simulink model "PIPO"  (R2024a)
settings: Solver=VariableStepAuto  StartTime=0.0  StopTime=10.0  RelTol=1e-3
libraries: simulink_extras x14
settings Model: Creator=prath  LastModifiedBy=prath

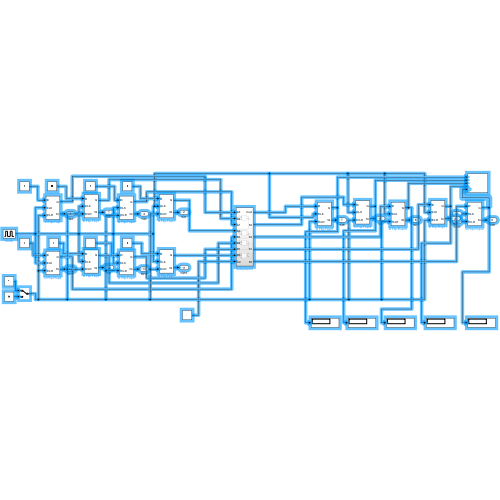
[thumbnail: Simulink's stored preview of the top-level diagram]
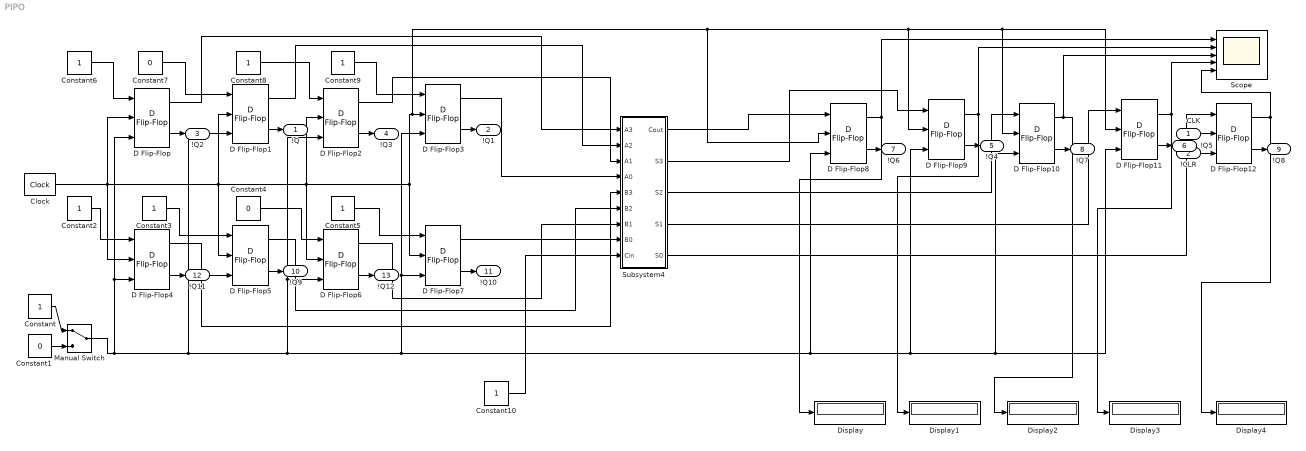
== system PIPO ==
  CLK : Inport
  !CLR : Inport  Port=2
  Clock : simulink_extras/Flip Flops/Clock  period=1
  Constant{,2..3,5..6,8..10} (8 alike) : Constant  OutDataTypeStr=boolean
  Constant1 : Constant  Value=0  OutDataTypeStr=boolean
  Constant4 : Constant  Value=0  OutDataTypeStr=boolean
  Constant7 : Constant  Value=0  OutDataTypeStr=boolean
  D Flip-Flop{,1..12} (13 alike) : simulink_extras/Flip Flops/D Flip-Flop
  Display{,1..4} (5 alike) : Display
  Manual Switch : ManualSwitch
  Scope : Scope  NumInputPorts=5
  Subsystem4 : Subsystem
  !Q : Outport
  !Q1 : Outport  Port=2
  !Q2 : Outport  Port=3
  !Q3 : Outport  Port=4
  !Q4 : Outport  Port=5
  !Q5 : Outport  Port=6
  !Q6 : Outport  Port=7
  !Q7 : Outport  Port=8
  !Q8 : Outport  Port=9
  !Q9 : Outport  Port=10
  !Q10 : Outport  Port=11
  !Q11 : Outport  Port=12
  !Q12 : Outport  Port=13
  wires:
  Subsystem4/5(S0) -> D Flip-Flop12/1
  D Flip-Flop/2 -> !Q2/1
  Constant/1 -> Manual Switch/1
  Constant7/1 -> D Flip-Flop1/1
  D Flip-Flop4/1 -> Subsystem4/5(B3)
  !CLR/1 -> D Flip-Flop12/3
  D Flip-Flop3/1 -> Subsystem4/4(A0)
  D Flip-Flop7/2 -> !Q10/1
  Constant8/1 -> D Flip-Flop2/1
  D Flip-Flop1/2 -> !Q/1
  D Flip-Flop/1 -> Subsystem4/1(A3)
  D Flip-Flop9/2 -> !Q4/1
  D Flip-Flop10/2 -> !Q7/1
  D Flip-Flop11/2 -> !Q5/1
  D Flip-Flop4/2 -> !Q11/1
  D Flip-Flop6/2 -> !Q12/1
  D Flip-Flop3/2 -> !Q1/1
  Constant5/1 -> D Flip-Flop7/1
  D Flip-Flop11/1 -> Scope/4, Display3/1
  Subsystem4/4(S1) -> D Flip-Flop11/1
  D Flip-Flop5/2 -> !Q9/1
  D Flip-Flop7/1 -> Subsystem4/8(B0)
  Subsystem4/1(Cout) -> D Flip-Flop8/1
  Constant9/1 -> D Flip-Flop3/1
  D Flip-Flop5/1 -> Subsystem4/6(B2)
  D Flip-Flop10/1 -> Scope/3, Display2/1
  Constant3/1 -> D Flip-Flop5/1
  D Flip-Flop1/1 -> Subsystem4/2(A2)
  CLK/1 -> D Flip-Flop12/2
  Constant4/1 -> D Flip-Flop6/1
  D Flip-Flop12/2 -> !Q8/1
  Subsystem4/3(S2) -> D Flip-Flop10/1
  D Flip-Flop8/1 -> Scope/1, Display/1
  D Flip-Flop8/2 -> !Q6/1
  Clock/1 -> D Flip-Flop4/2, D Flip-Flop/2, D Flip-Flop5/2, D Flip-Flop1/2, D Flip-Flop2/2, D Flip-Flop6/2, D Flip-Flop8/2, D Flip-Flop9/2, D Flip-Flop10/2, D Flip-Flop11/2, D Flip-Flop3/2, D Flip-Flop7/2
  Subsystem4/2(S3) -> D Flip-Flop9/1
  Constant2/1 -> D Flip-Flop4/1
  D Flip-Flop9/1 -> Scope/2, Display1/1
  Manual Switch/1 -> D Flip-Flop4/3, D Flip-Flop/3, D Flip-Flop5/3, D Flip-Flop1/3, D Flip-Flop2/3, D Flip-Flop6/3, D Flip-Flop8/3, D Flip-Flop9/3, D Flip-Flop10/3, D Flip-Flop11/3, D Flip-Flop7/3, D Flip-Flop3/3
  D Flip-Flop2/1 -> Subsystem4/3(A1)
  D Flip-Flop6/1 -> Subsystem4/7(B1)
  Constant6/1 -> D Flip-Flop/1
  Constant10/1 -> Subsystem4/9(Cin)
  Constant1/1 -> Manual Switch/2
  D Flip-Flop2/2 -> !Q3/1
  D Flip-Flop12/1 -> Scope/5, Display4/1

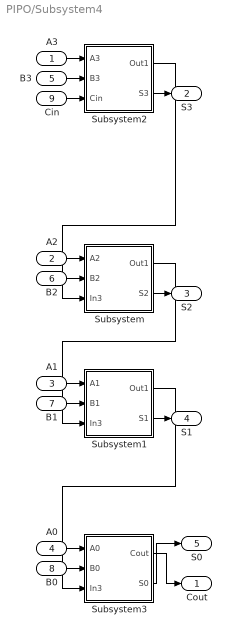
== system PIPO/Subsystem4 ==
  A3 : Inport
  A2 : Inport  Port=2
  A1 : Inport  Port=3
  A0 : Inport  Port=4
  B3 : Inport  Port=5
  B2 : Inport  Port=6
  B1 : Inport  Port=7
  B0 : Inport  Port=8
  Cin : Inport  Port=9
  Subsystem : Subsystem
  Subsystem1 : Subsystem
  Subsystem2 : Subsystem
  Subsystem3 : Subsystem
  Cout : Outport
  S3 : Outport  Port=2
  S2 : Outport  Port=3
  S1 : Outport  Port=4
  S0 : Outport  Port=5
  wires:
  Subsystem2/1(Out1) -> Subsystem/3(In3)
  Subsystem2/2(S3) -> S3/1
  B0/1 -> Subsystem3/2(B0)
  Subsystem1/1(Out1) -> Subsystem3/3(In3)
  Subsystem/1(Out1) -> Subsystem1/3(In3)
  Subsystem3/2(S0) -> S0/1
  A2/1 -> Subsystem/1(A2)
  Subsystem/2(S2) -> S2/1
  A0/1 -> Subsystem3/1(A0)
  B1/1 -> Subsystem1/2(B1)
  Subsystem3/1(Cout) -> Cout/1
  B2/1 -> Subsystem/2(B2)
  B3/1 -> Subsystem2/2(B3)
  Cin/1 -> Subsystem2/3(Cin)
  Subsystem1/2(S1) -> S1/1
  A3/1 -> Subsystem2/1(A3)
  A1/1 -> Subsystem1/1(A1)

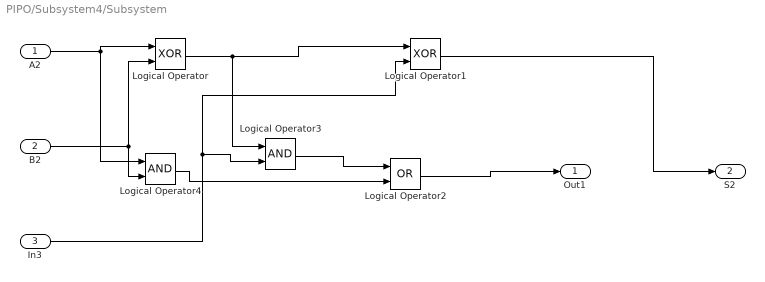
== system PIPO/Subsystem4/Subsystem ==
  A2 : Inport
  B2 : Inport  Port=2
  In3 : Inport  Port=3
  Logical Operator : Logic  Operator=XOR  AllPortsSameDT=off  OutDataTypeStr=boolean
  Logical Operator1 : Logic  Operator=XOR  AllPortsSameDT=off  OutDataTypeStr=boolean
  Logical Operator2 : Logic  Operator=OR  AllPortsSameDT=off  OutDataTypeStr=boolean
  Logical Operator3 : Logic  AllPortsSameDT=off  OutDataTypeStr=boolean
  Logical Operator4 : Logic  AllPortsSameDT=off  OutDataTypeStr=boolean
  Out1 : Outport
  S2 : Outport  Port=2
  wires:
  B2/1 -> Logical Operator/2, Logical Operator4/2
  Logical Operator/1 -> Logical Operator3/1, Logical Operator1/1
  In3/1 -> Logical Operator3/2, Logical Operator1/2
  Logical Operator3/1 -> Logical Operator2/1
  Logical Operator2/1 -> Out1/1
  A2/1 -> Logical Operator/1, Logical Operator4/1
  Logical Operator4/1 -> Logical Operator2/2
  Logical Operator1/1 -> S2/1

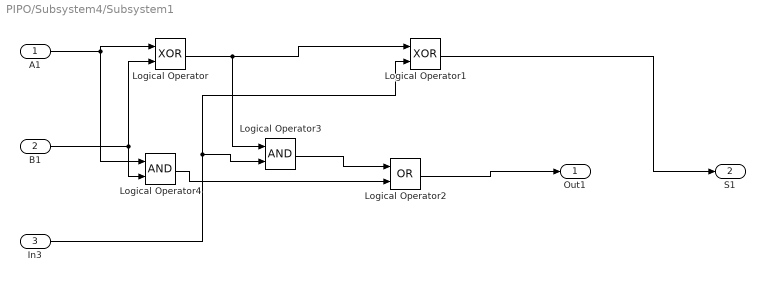
== system PIPO/Subsystem4/Subsystem1 ==
  A1 : Inport
  B1 : Inport  Port=2
  In3 : Inport  Port=3
  Logical Operator : Logic  Operator=XOR  AllPortsSameDT=off  OutDataTypeStr=boolean
  Logical Operator1 : Logic  Operator=XOR  AllPortsSameDT=off  OutDataTypeStr=boolean
  Logical Operator2 : Logic  Operator=OR  AllPortsSameDT=off  OutDataTypeStr=boolean
  Logical Operator3 : Logic  AllPortsSameDT=off  OutDataTypeStr=boolean
  Logical Operator4 : Logic  AllPortsSameDT=off  OutDataTypeStr=boolean
  Out1 : Outport
  S1 : Outport  Port=2
  wires:
  B1/1 -> Logical Operator/2, Logical Operator4/2
  Logical Operator/1 -> Logical Operator3/1, Logical Operator1/1
  In3/1 -> Logical Operator3/2, Logical Operator1/2
  Logical Operator3/1 -> Logical Operator2/1
  Logical Operator2/1 -> Out1/1
  A1/1 -> Logical Operator/1, Logical Operator4/1
  Logical Operator4/1 -> Logical Operator2/2
  Logical Operator1/1 -> S1/1

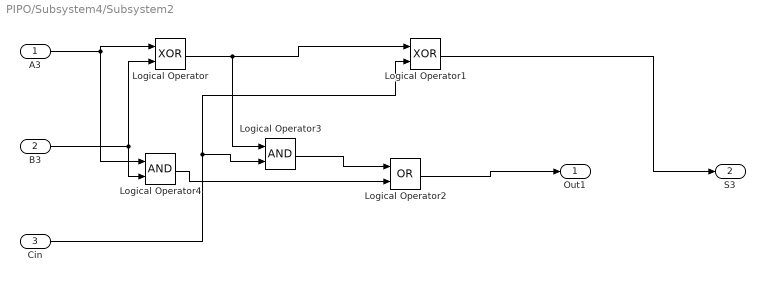
== system PIPO/Subsystem4/Subsystem2 ==
  A3 : Inport
  B3 : Inport  Port=2
  Cin : Inport  Port=3
  Logical Operator : Logic  Operator=XOR  AllPortsSameDT=off  OutDataTypeStr=boolean
  Logical Operator1 : Logic  Operator=XOR  AllPortsSameDT=off  OutDataTypeStr=boolean
  Logical Operator2 : Logic  Operator=OR  AllPortsSameDT=off  OutDataTypeStr=boolean
  Logical Operator3 : Logic  AllPortsSameDT=off  OutDataTypeStr=boolean
  Logical Operator4 : Logic  AllPortsSameDT=off  OutDataTypeStr=boolean
  Out1 : Outport
  S3 : Outport  Port=2
  wires:
  B3/1 -> Logical Operator/2, Logical Operator4/2
  Logical Operator/1 -> Logical Operator3/1, Logical Operator1/1
  Cin/1 -> Logical Operator3/2, Logical Operator1/2
  Logical Operator3/1 -> Logical Operator2/1
  Logical Operator2/1 -> Out1/1
  A3/1 -> Logical Operator/1, Logical Operator4/1
  Logical Operator4/1 -> Logical Operator2/2
  Logical Operator1/1 -> S3/1

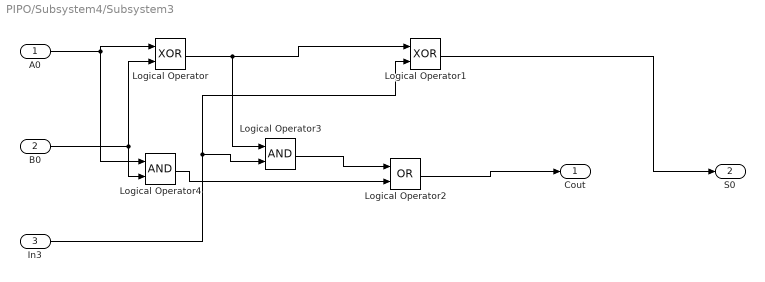
== system PIPO/Subsystem4/Subsystem3 ==
  A0 : Inport
  B0 : Inport  Port=2
  In3 : Inport  Port=3
  Logical Operator : Logic  Operator=XOR  AllPortsSameDT=off  OutDataTypeStr=boolean
  Logical Operator1 : Logic  Operator=XOR  AllPortsSameDT=off  OutDataTypeStr=boolean
  Logical Operator2 : Logic  Operator=OR  AllPortsSameDT=off  OutDataTypeStr=boolean
  Logical Operator3 : Logic  AllPortsSameDT=off  OutDataTypeStr=boolean
  Logical Operator4 : Logic  AllPortsSameDT=off  OutDataTypeStr=boolean
  Cout : Outport
  S0 : Outport  Port=2
  wires:
  B0/1 -> Logical Operator/2, Logical Operator4/2
  Logical Operator/1 -> Logical Operator3/1, Logical Operator1/1
  In3/1 -> Logical Operator3/2, Logical Operator1/2
  Logical Operator3/1 -> Logical Operator2/1
  Logical Operator2/1 -> Cout/1
  A0/1 -> Logical Operator/1, Logical Operator4/1
  Logical Operator4/1 -> Logical Operator2/2
  Logical Operator1/1 -> S0/1
